simulink model "iterative_rigid"  (R2021b)
settings: Solver=VariableStepAuto  StartTime=0.0  StopTime=30.0  RelTol=1e-3
undefined symbols (not defined in the file): Kd, Kp, qd
libraries: simulink x1
settings Model: Creator=fabioscap  LastModifiedBy=fabioscap

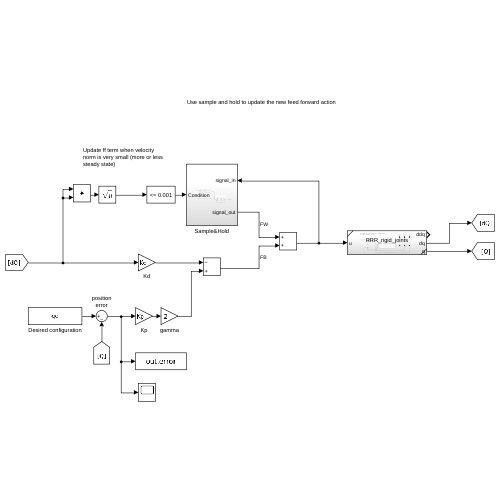
[thumbnail: Simulink's stored preview of the top-level diagram]
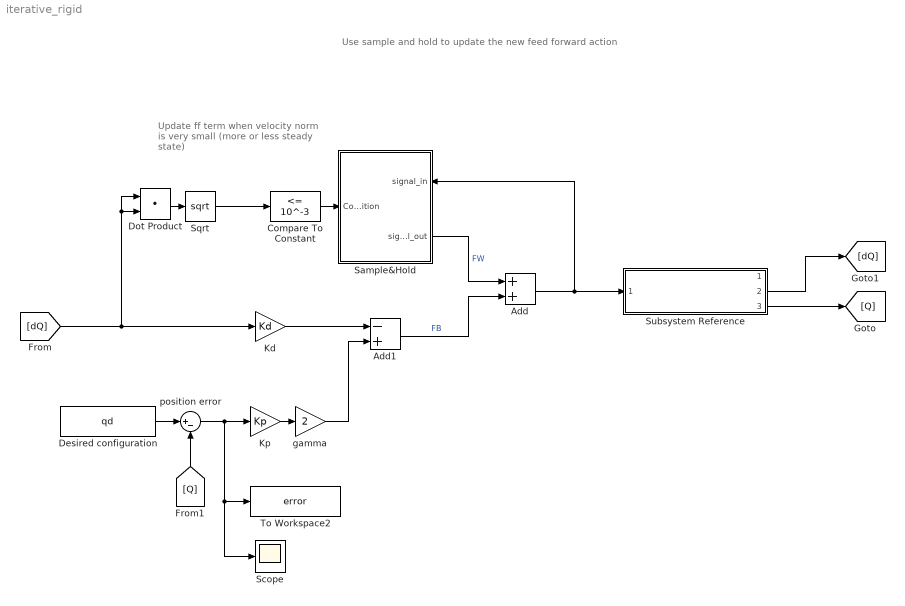
== system iterative_rigid ==
  note: Update ff term when velocity norm is very small (more or less steady state)
  note: Use sample and hold to update the new feed forward action
  Add : Sum
  Add1 : Sum  Inputs=-+
  Compare To Constant : simulink/Logic and Bit Operations/Compare To Constant  relop=<=  const=10^-3  OutDataTypeStr=boolean
  Desired configuration : Constant  Value=qd
  Dot Product : DotProduct  InputSameDT=on  OutDataTypeStr=Inherit: Inherit via internal rule
  Kd : Gain  Gain=Kd
  Kp : Gain  Gain=Kp
  Sample&Hold : Subsystem
      settings: PortSchema="{\"entries\":[{\"content\":{\"sides\":[{\"content\":{\"connectorIds\":[\"In1\"]},\"type\":\"ConnectorPlacement.EquallySpacedRectSide\",\"uuid\":\"4e144169-49b5-4e4c-b5f4-9ef7c3f2f0f9\"},{\"content\":{\"connectorIds\":[\"In2\",\"Out1\"],\"side\":\"RIGHT\"},\"type\":\"ConnectorPlacement.EquallySpacedRectSide\",\"uuid\":\"f363b949-3911-4beb-ab4e-918606327600\"},{\"content\":{\"connectorIds\":[],\"side\":\"TOP\"},\"type\":\"ConnectorPlacement.EquallySpacedRectSide\",\"uuid\":\"9c880683-fb68-40e9-87c7-4f0e0baabf9f\"}]},\"type\":\"ConnectorPlacement.EquallySpacedConnector\",\"uuid\":\"d3c18749-4c54-4ed6-af1e-c9020595430a\"}],\"packageUris\":[\"http://schema.mathworks.com/mf0/Connector/R2020b\"],\"version\":\"1.0\"}"
  Scope : Scope
  Sqrt : Sqrt  SaturateOnIntegerOverflow=on
  Subsystem Reference : Subsystem  ReferencedSubsystem=RRR_rigid_joints
  To Workspace2 : ToWorkspace  VariableName=error  SaveFormat=Timeseries  SampleTime=-1
  gamma : Gain  Gain=2
  position error : Sum  Inputs=|+-
  wires:
  Add/1 -> Subsystem Reference/1, Sample&Hold/2(signal_in)
  Sample&Hold/1(signal_out) -> Add/1  "FW"
  position error/1 -> Scope/1, To Workspace2/1, Kp/1
  Desired configuration/1 -> position error/1
  Kd/1 -> Add1/1
  Add1/1 -> Add/2  "FB"
  Subsystem Reference/3 -> [Q]
  Subsystem Reference/2 -> [dQ]
  [Q] -> position error/2
  Kp/1 -> gamma/1
  gamma/1 -> Add1/2
  [dQ] -> Dot Product/1, Dot Product/2, Kd/1
  Compare To Constant/1 -> Sample&Hold/1(Condition)
  Dot Product/1 -> Sqrt/1
  Sqrt/1 -> Compare To Constant/1

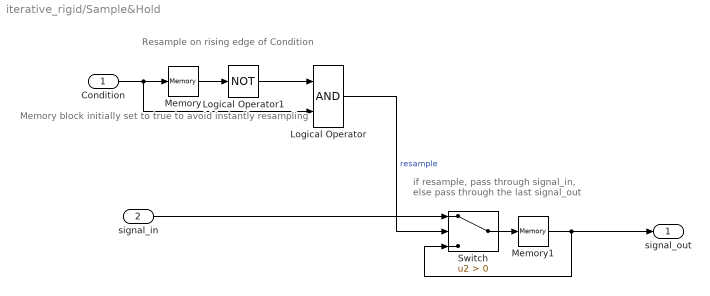
== system iterative_rigid/Sample&Hold ==
  note: Memory block initially set to true to avoid instantly resampling
  note: if resample, pass through signal_in,
      | else pass through the last signal_out
  note: Resample on rising edge of Condition
  Condition : Inport
  signal_in : Inport  Port=2
  Logical Operator : Logic  AllPortsSameDT=off  OutDataTypeStr=boolean
  Logical Operator1 : Logic  Operator=NOT  AllPortsSameDT=off  OutDataTypeStr=boolean
  Memory : Memory  InitialCondition=1
  Memory1 : Memory
  Switch : Switch  Criteria=u2 > Threshold
  signal_out : Outport
  wires:
  Condition/1 -> Logical Operator/2, Memory/1
  Memory/1 -> Logical Operator1/1
  Logical Operator1/1 -> Logical Operator/1
  signal_in/1 -> Switch/1
  Logical Operator/1 -> Switch/2  "resample"
  Memory1/1 -> Switch/3, signal_out/1
  Switch/1 -> Memory1/1
